simulink model "ftemp"  (R2019a)
settings: Solver=VariableStepAuto  StartTime=0.0  StopTime=10.0  RelTol=1e-3
libraries: nesl_utility x4, fl_lib x1
settings Model: Creator=karth  LastModifiedBy=karth

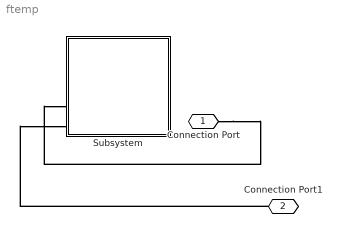
== system ftemp ==
  Subsystem : Subsystem
  Connection Port : PMIOPort  Side=Left
  Connection Port1 : PMIOPort  Port=2  Side=Left
  connections:
  Connection Port/RConn1 -- Subsystem/LConn4
  Connection Port1/RConn1 -- Subsystem/LConn5

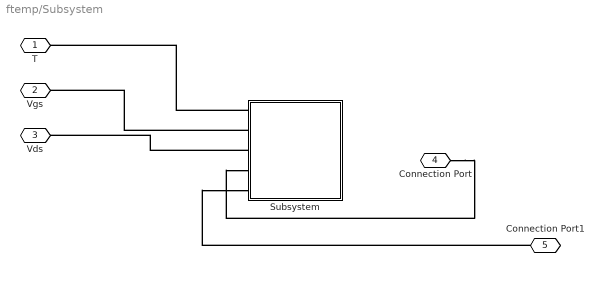
== system ftemp/Subsystem ==
  Subsystem : Subsystem
  T : PMIOPort  Side=Left
  Vgs : PMIOPort  Port=2  Side=Left
  Vds : PMIOPort  Port=3  Side=Left
  Connection Port : PMIOPort  Port=4  Side=Left
  Connection Port1 : PMIOPort  Port=5  Side=Left
  connections:
  Subsystem/LConn1 -- T/RConn1
  Subsystem/LConn2 -- Vgs/RConn1
  Subsystem/LConn3 -- Vds/RConn1
  Connection Port/RConn1 -- Subsystem/LConn4
  Connection Port1/RConn1 -- Subsystem/LConn5

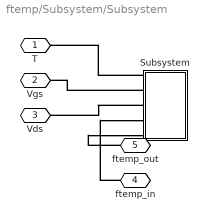
== system ftemp/Subsystem/Subsystem ==
  Subsystem : Subsystem
  T : PMIOPort  Side=Left
  Vgs : PMIOPort  Port=2  Side=Left
  Vds : PMIOPort  Port=3  Side=Left
  ftemp_in : PMIOPort  Port=4  Side=Left
  ftemp_out : PMIOPort  Port=5  Side=Left
  connections:
  Subsystem/LConn1 -- T/RConn1
  Subsystem/LConn2 -- Vgs/RConn1
  Subsystem/LConn3 -- Vds/RConn1
  ftemp_in/RConn1 -- Subsystem/LConn4
  ftemp_out/RConn1 -- Subsystem/LConn5

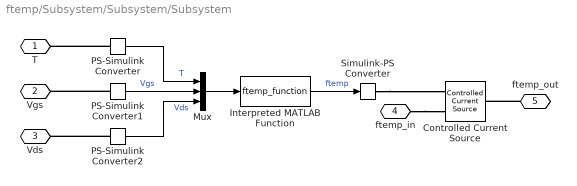
== system ftemp/Subsystem/Subsystem/Subsystem ==
  Controlled Current Source : fl_lib/Electrical/Electrical Sources/Controlled Current Source
  Interpreted MATLAB Function : MATLABFcn  MATLABFcn=ftemp_function
  Mux : Mux  Inputs=3
  PS-Simulink Converter : nesl_utility/PS-Simulink Converter  PhysicalDomain=network_engine_domain  SubClassName=ps_output  LeftPortType=input  RightPortType=output  PseudoPeriodic=off  Frequencies=[]  Unit=1  AffineConversion=off
  PS-Simulink Converter1 : nesl_utility/PS-Simulink Converter  PhysicalDomain=network_engine_domain  SubClassName=ps_output  LeftPortType=input  RightPortType=output  PseudoPeriodic=off  Frequencies=[]  Unit=1  AffineConversion=off
  PS-Simulink Converter2 : nesl_utility/PS-Simulink Converter  PhysicalDomain=network_engine_domain  SubClassName=ps_output  LeftPortType=input  RightPortType=output  PseudoPeriodic=off  Frequencies=[]  Unit=1  AffineConversion=off
  Simulink-PS Converter : nesl_utility/Simulink-PS Converter  PhysicalDomain=network_engine_domain  SubClassName=ps_input  LeftPortType=input  RightPortType=output  PseudoPeriodic=off  Frequencies=[]  NoiseDistribution=none  NoiseParameters=[]  Unit=1  AffineConversion=off  FilteringAndDerivatives=provide  SimscapeFilterOrder=1  InputFilterTimeConstant=0.001  UdotUserProvided=0
  T : PMIOPort  Side=Left
  Vgs : PMIOPort  Port=2  Side=Left
  Vds : PMIOPort  Port=3  Side=Left
  ftemp_in : PMIOPort  Port=4  Side=Left
  ftemp_out : PMIOPort  Port=5  Side=Left
  wires:
  Interpreted MATLAB Function/1 -> Simulink-PS Converter/1  "ftemp"
  PS-Simulink Converter2/1 -> Mux/3  "Vds"
  PS-Simulink Converter1/1 -> Mux/2  "Vgs"
  PS-Simulink Converter/1 -> Mux/1  "T"
  Mux/1 -> Interpreted MATLAB Function/1
  connections:
  ftemp_in/RConn1 -- Controlled Current Source/RConn2
  PS-Simulink Converter2/LConn1 -- Vds/RConn1
  PS-Simulink Converter1/LConn1 -- Vgs/RConn1
  Simulink-PS Converter/RConn1 -- Controlled Current Source/RConn1
  PS-Simulink Converter/LConn1 -- T/RConn1
  ftemp_out/RConn1 -- Controlled Current Source/LConn1
